simulink model "inverse_GSFR_Individual_Vars"  (R2019b)
settings: Solver=VariableStepAuto  StartTime=0.0  StopTime=20  MaxStep=0.01  RelTol=1e-3
values from neighbouring files (symbols this model uses):
  a1 = (D*R+K)*2*c*wn    [Injections_plot.m]    (also in Monte_Carlo_GSFR_Half_Length_Injection.m; Monte_Carlo_GSFR_Ideal_Injection.m; Monte_Carlo_GSFR_Simplified_Injection.m; dpt_from_dft_H.m)
  b1 = wn^2    [Injections_plot.m]    (also in Monte_Carlo_GSFR_Half_Length_Injection.m; Monte_Carlo_GSFR_Ideal_Injection.m; Monte_Carlo_GSFR_Simplified_Injection.m; dpt_from_dft_H.m)
  c = (((2*H*R)+(((D*R)+(K*Fh))*Tr))/(2*(D*R+K)))*wn    [Injections_plot.m]    (also in Monte_Carlo_GSFR_Half_Length_Injection.m; Monte_Carlo_GSFR_Ideal_Injection.m; Monte_Carlo_GSFR_Simplified_Injection.m; dpt_from_dft_H.m)
  c1 = (wn^2)*R*Tr    [Injections_plot.m]    (also in Monte_Carlo_GSFR_Half_Length_Injection.m; Monte_Carlo_GSFR_Ideal_Injection.m; Monte_Carlo_GSFR_Simplified_Injection.m; dpt_from_dft_H.m)
  D = 1.0    (= 1)    [Injections_plot.m]    (also in Monte_Carlo_GSFR_Half_Length_Injection.m; Monte_Carlo_GSFR_Ideal_Injection.m; Monte_Carlo_GSFR_Simplified_Injection.m; dpt_from_dft_H.m)
  d1 = (wn^2)*R    [Injections_plot.m]    (also in Monte_Carlo_GSFR_Half_Length_Injection.m; Monte_Carlo_GSFR_Ideal_Injection.m; Monte_Carlo_GSFR_Simplified_Injection.m; dpt_from_dft_H.m)
  K = 0.95    [Injections_plot.m]    (also in Monte_Carlo_GSFR_Half_Length_Injection.m; Monte_Carlo_GSFR_Ideal_Injection.m; Monte_Carlo_GSFR_Simplified_Injection.m; dpt_from_dft_H.m)
  R = 0.075    [Injections_plot.m]    (also in Monte_Carlo_GSFR_Half_Length_Injection.m = (0.05/3)*randn()+0.075; Monte_Carlo_GSFR_Ideal_Injection.m = (0.05/3)*randn()+0.075; Monte_Carlo_GSFR_Simplified_Injection.m = (0.05/3)*randn()+0.075; dpt_from_dft_H.m = 0.05)
  Tr = 9.0    (= 9)    [Injections_plot.m]    (also in Monte_Carlo_GSFR_Half_Length_Injection.m = 0.67*randn()+9; Monte_Carlo_GSFR_Ideal_Injection.m = 0.67*randn()+9; Monte_Carlo_GSFR_Simplified_Injection.m = 0.67*randn()+9; dpt_from_dft_H.m = 8)
  wn = sqrt((D*R+K)/(2*H*R*Tr))    [Injections_plot.m]    (also in Monte_Carlo_GSFR_Half_Length_Injection.m; Monte_Carlo_GSFR_Ideal_Injection.m; Monte_Carlo_GSFR_Simplified_Injection.m; dpt_from_dft_H.m)
  x1 = D*R+K    (= 1.025)    [Injections_plot.m]    (also in Monte_Carlo_GSFR_Half_Length_Injection.m; Monte_Carlo_GSFR_Ideal_Injection.m; Monte_Carlo_GSFR_Simplified_Injection.m; dpt_from_dft_H.m = 1)
settings Model: Creator=ruiva  LastModifiedBy=ruiva

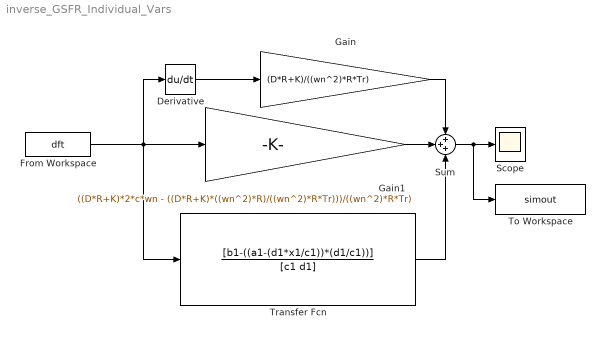
== system inverse_GSFR_Individual_Vars ==
  Derivative : Derivative
  From Workspace : FromWorkspace  VariableName=dft  SampleTime=0
  Gain : Gain  Gain=(D*R+K)/((wn^2)*R*Tr)
  Gain1 : Gain  Gain=((D*R+K)*2*c*wn - ((D*R+K)*((wn^2)*R)/((wn^2)*R*Tr)))/((wn^2)*R*Tr)
  Scope : Scope
  Sum : Sum  Inputs=+++
  To Workspace : ToWorkspace  VariableName=simout  SaveFormat=Timeseries  SampleTime=-1
  Transfer Fcn : TransferFcn  Numerator=[b1-((a1-(d1*x1/c1))*(d1/c1))]  Denominator=[c1 d1]
  wires:
  Derivative/1 -> Gain/1
  From Workspace/1 -> Transfer Fcn/1, Gain1/1, Derivative/1
  Transfer Fcn/1 -> Sum/3
  Gain1/1 -> Sum/2
  Gain/1 -> Sum/1
  Sum/1 -> To Workspace/1, Scope/1
